simulink model "calkowanie"  (R2022b)
settings: Solver=VariableStepAuto  StartTime=0.0  StopTime=10.0  RelTol=1e-3
values from neighbouring files (symbols this model uses):
  B = B .* 1.8    [dodatkowe.m]
  Kexp = acker(Aexp, Bexp, [sc, sc, sc, sc])    [dodatkowe.m]
settings Model: Creator=antekgrajek  LastModifiedBy=antekgrajek

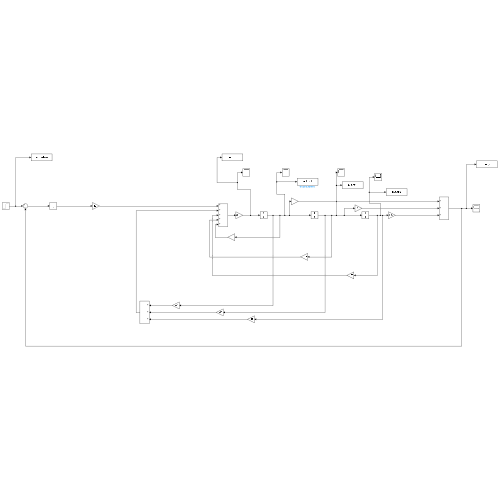
[thumbnail: Simulink's stored preview of the top-level diagram]
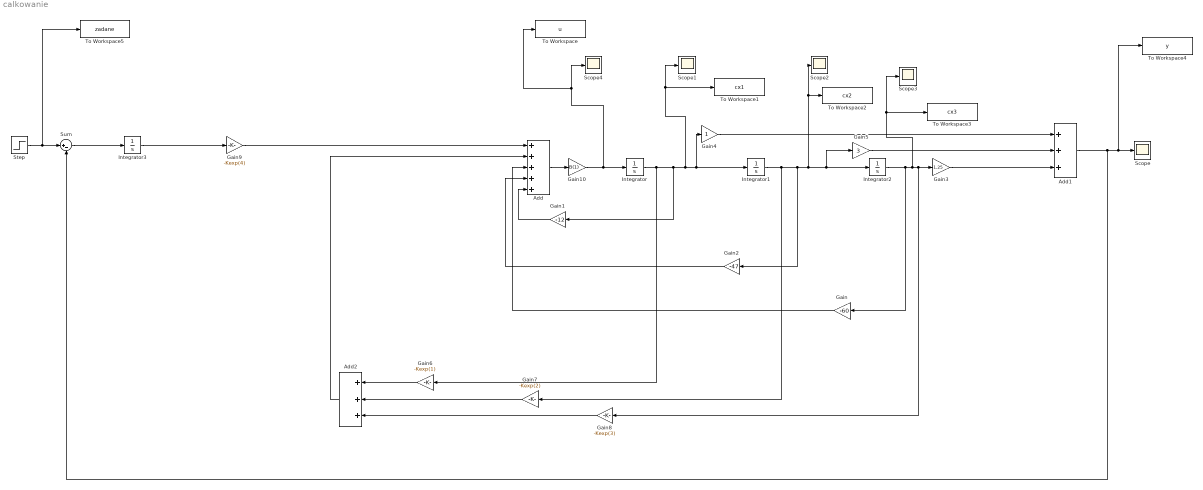
== system calkowanie ==
  Add : Sum  Inputs=+++++
  Add1 : Sum  Inputs=+++
  Add2 : Sum  Inputs=+++
  Gain : Gain  Gain=-60
  Gain1 : Gain  Gain=-12
  Gain10 : Gain  Gain=B(1)
  Gain2 : Gain  Gain=-47
  Gain3 : Gain  Gain=1.25
  Gain4 : Gain
  Gain5 : Gain  Gain=3
  Gain6 : Gain  Gain=-Kexp(1)
  Gain7 : Gain  Gain=-Kexp(2)
  Gain8 : Gain  Gain=-Kexp(3)
  Gain9 : Gain  Gain=-Kexp(4)
  Integrator : Integrator  InitialCondition=5
  Integrator1 : Integrator  InitialCondition=6
  Integrator2 : Integrator  InitialCondition=1
  Integrator3 : Integrator  InitialCondition=5
  Scope{,1..4} (5 alike) : Scope
  Step : Step  After=5  SampleTime=0
  Sum : Sum  Inputs=|+-
  To Workspace : ToWorkspace  VariableName=u  SaveFormat=Timeseries  SampleTime=-1
  To Workspace1 : ToWorkspace  VariableName=cx1  SaveFormat=Timeseries  SampleTime=-1
  To Workspace2 : ToWorkspace  VariableName=cx2  SaveFormat=Timeseries  SampleTime=-1
  To Workspace3 : ToWorkspace  VariableName=cx3  SaveFormat=Timeseries  SampleTime=-1
  To Workspace4 : ToWorkspace  VariableName=y  SaveFormat=Timeseries  SampleTime=-1
  To Workspace5 : ToWorkspace  VariableName=zadane  SaveFormat=Timeseries  SampleTime=-1
  wires:
  Integrator2/1 -> Gain/1, To Workspace3/1, Scope3/1, Gain8/1, Gain3/1
  Gain4/1 -> Add1/1
  Gain6/1 -> Add2/1
  Gain5/1 -> Add1/2
  Gain2/1 -> Add/4
  Gain/1 -> Add/3
  Add2/1 -> Add/2
  Integrator1/1 -> Gain7/1, Gain2/1, To Workspace2/1, Scope2/1, Gain5/1, Integrator2/1
  Gain1/1 -> Add/5
  Gain8/1 -> Add2/3
  Integrator/1 -> Gain6/1, Gain1/1, To Workspace1/1, Scope1/1, Gain4/1, Integrator1/1
  Gain7/1 -> Add2/2
  Gain3/1 -> Add1/3
  Integrator3/1 -> Gain9/1
  Gain9/1 -> Add/1
  Add1/1 -> Sum/2, To Workspace4/1, Scope/1
  Sum/1 -> Integrator3/1
  Step/1 -> To Workspace5/1, Sum/1
  Add/1 -> Gain10/1
  Gain10/1 -> To Workspace/1, Scope4/1, Integrator/1
